simulink model "work1"  (R2020b)
settings: Solver=VariableStepAuto  StartTime=0.0  StopTime=10.0  RelTol=1e-3
settings Model: Creator=99003178  LastModifiedBy=99003178

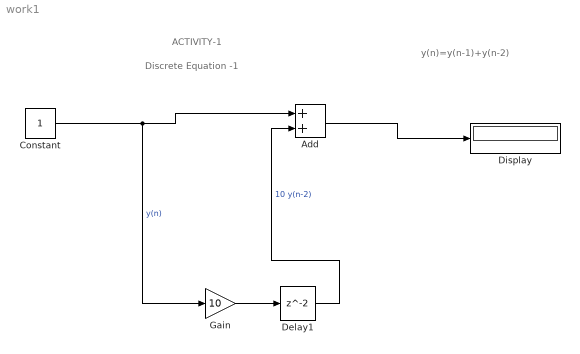
== system work1 ==
  note: Discrete Equation -1
  note: ACTIVITY-1
  note: y(n)=y(n-1)+y(n-2)
  Add : Sum
  Constant : Constant
  Delay1 : Delay
  Display : Display
  Gain : Gain  Gain=10
  wires:
  Constant/1 -> Gain/1, Add/1  "y(n)"
  Add/1 -> Display/1
  Gain/1 -> Delay1/1
  Delay1/1 -> Add/2  "10 y(n-2)"
